simulink model "NES"  (R2024b)
settings: Solver=VariableStepAuto  StartTime=0.0  StopTime=10.0  RelTol=1e-3
settings Model: Creator=quinn  LastModifiedBy=quinn

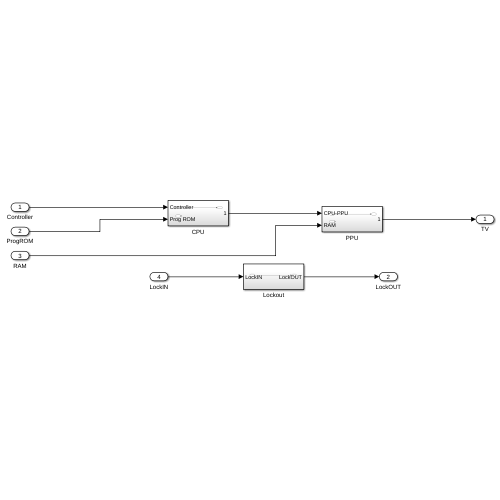
[thumbnail: Simulink's stored preview of the top-level diagram]
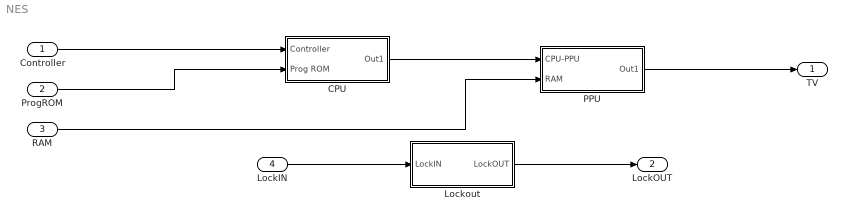
== system NES ==
  Controller : Inport
  ProgROM : Inport  Port=2
  RAM : Inport  Port=3
  LockIN : Inport  Port=4
  CPU : Subsystem
  Lockout : Subsystem
  PPU : Subsystem
  TV : Outport
  LockOUT : Outport  Port=2
  wires:
  Controller/1 -> CPU/1(Controller)
  CPU/1(Out1) -> PPU/1(CPU-PPU)
  PPU/1(Out1) -> TV/1
  Lockout/1(LockOUT) -> LockOUT/1
  LockIN/1 -> Lockout/1(LockIN)
  ProgROM/1 -> CPU/2(Prog ROM)
  RAM/1 -> PPU/2(RAM)

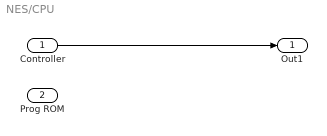
== system NES/CPU ==
  Controller : Inport
  Prog ROM : Inport  Port=2
  Out1 : Outport
  wires:
  Controller/1 -> Out1/1

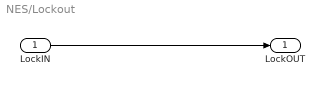
== system NES/Lockout ==
  LockIN : Inport
  LockOUT : Outport
  wires:
  LockIN/1 -> LockOUT/1

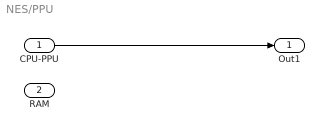
== system NES/PPU ==
  CPU-PPU : Inport
  RAM : Inport  Port=2
  Out1 : Outport
  wires:
  CPU-PPU/1 -> Out1/1
